simulink model "Dynamic_articulation_FSFA"  (R2018b)
settings: Solver=VariableStepAuto  StartTime=0.0  StopTime=t_final  RelTol=1e-9
values from neighbouring files (symbols this model uses):
  a2 = input(12)    [Nonlinear_model.m]    (also in linear_model.m; linear_model_error.m; trailer_constants.m = 4.98)
  Am = [-0.5 0 0 0 0 0 0 0 ... (first row only)    [Dynamic_model_articulation.m]
  Ap = A    [Dynamic_model_articulation.m]    (also in articulation.m = -1*M_inv*K/u)
  Aprime = A - B1*K    [Dynamic_model_articulation.m]
  B1 = [0,B1(1),0,B1(2),0,B1(3),0,B1(4)]'    [articulation1.m]
  B2 = [0,B2(1),0,B2(2),0,B2(3),0,B2(4)]'    [articulation1.m]
  Bm = [1;0;0;0]    [Dynamic_model_articulation.m]
  Bm2 = B2    [Dynamic_model_articulation.m]
  constants = [C1 C2 C3 m1 m2 I1 I2 a1 l1 h1 b1 a2 l2 Vx]    [Dynamic_model_articulation.m]
  h1 = input(10)    [Nonlinear_model.m]    (also in linear_model.m; linear_model_error.m; truck_constants.m = 1.1)
  K = place(A,B1,Poles)    [FullStateFeedback.m]    (also in articulation.m = [(C+C3),     (Cs1-C3*(h1+l2)+(m1+m2)*u^2),    (-C3*l2),    (; articulation1.m = [(C+C3),     (Cs1-C3*(h1+l2)+(m1+m2)*u^2),    (-C3*l2),    (; linear_model.m = -1/u*K*x_bar; linear_model_error.m = -1/u*K*x_bar)
  Lamda = 0.03    [Dynamic_model_articulation.m]
  Pm = lyap(Am,Q)    [Dynamic_model_articulation.m]
  Vx = 20    [Dynamic_model_articulation.m]
settings Model: Creator=kevingasik  LastModifiedBy=kevingasik
settings DataIOCC: OutputOption=SpecifiedOutputTimes  OutputTimes=[0:0.04:t_final]

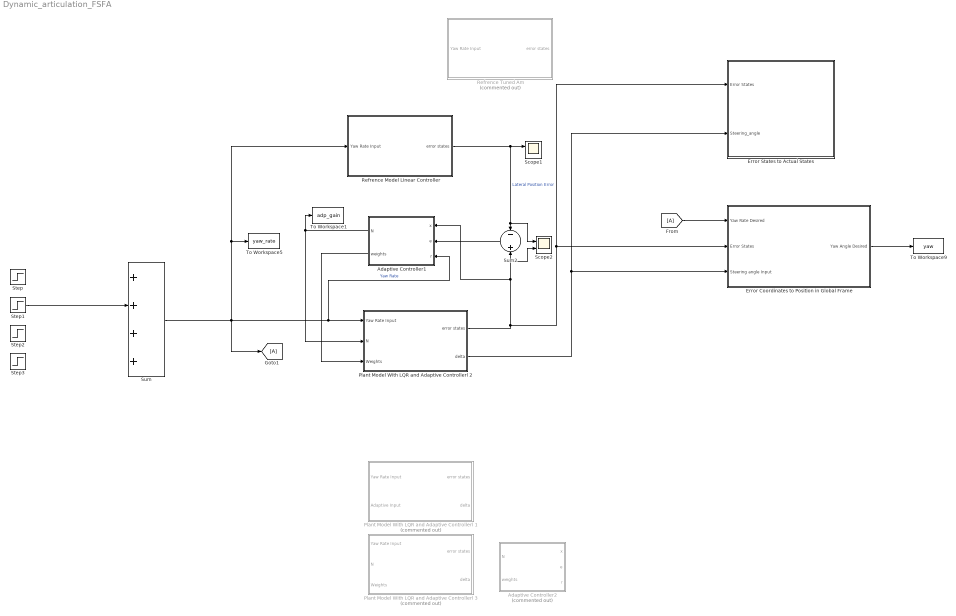
== system Dynamic_articulation_FSFA ==
  Adaptive Controller1 : Subsystem
  Adaptive Controller2 : Subsystem  Commented=on
  "Error Coordinates to Position in Global Frame " : Subsystem
  Error States to Actual States : Subsystem
  Plant Model With LQR and Adaptive Controllerl 1 : Subsystem  Commented=on
  Plant Model With LQR and Adaptive Controllerl 2 : Subsystem
  Plant Model With LQR and Adaptive Controllerl 3 : Subsystem  Commented=on
  Refrence Model Linear Controller : Subsystem
  Refrence Tuned Am : Subsystem  Commented=on
  Scope1 : Scope  NumInputPorts=2
  Scope2 : Scope  NumInputPorts=2
  Step : Step  Time=0  After=0  SampleTime=0
  Step1 : Step  Time=0  After=0.5/180*pi  SampleTime=0
  Step2 : Step  Time=200  After=-1/180*pi  SampleTime=0
  Step3 : Step  Time=110  After=0.5/180*pi  SampleTime=0
  Sum : Sum  Inputs=++++
  Sum2 : Sum  Inputs=-+
  To Workspace1 : ToWorkspace  VariableName=adp_gain  SampleTime=-1
      settings: Save2DSignal=2-D array (concatenate along first dimension)
  To Workspace5 : ToWorkspace  VariableName=yaw_rate  SampleTime=-1
      settings: Save2DSignal=2-D array (concatenate along first dimension)
  To Workspace9 : ToWorkspace  VariableName=yaw  SampleTime=-1
      settings: Save2DSignal=2-D array (concatenate along first dimension)
  wires:
  Sum/1 -> Adaptive Controller1/3(r), Plant Model With LQR and Adaptive Controllerl 2/1(Yaw Rate Input), Refrence Model Linear Controller/1(Yaw Rate Input), To Workspace5/1, [A]  "Yaw Rate"
  Plant Model With LQR and Adaptive Controllerl 2/1(error states) -> "Error Coordinates to Position in Global Frame "/2(Error States), Error States to Actual States/1(Error States), Adaptive Controller1/1(x), Scope2/2, Sum2/2
  Sum2/1 -> Adaptive Controller1/2(e)
  Step1/1 -> Sum/2
  Adaptive Controller1/1(N) -> Plant Model With LQR and Adaptive Controllerl 2/2(N), To Workspace1/1
  [A] -> "Error Coordinates to Position in Global Frame "/1(Yaw Rate Desired)
  Plant Model With LQR and Adaptive Controllerl 2/2(delta) -> Error States to Actual States/2(Steering_angle), "Error Coordinates to Position in Global Frame "/3(Steering angle Input)
  "Error Coordinates to Position in Global Frame "/1(Yaw Angle Desired) -> To Workspace9/1
  Refrence Model Linear Controller/1(error states) -> Scope2/1, Sum2/1, Scope1/1  "Lateral Position Error"
  Adaptive Controller1/2(weights) -> Plant Model With LQR and Adaptive Controllerl 2/3(Weights)

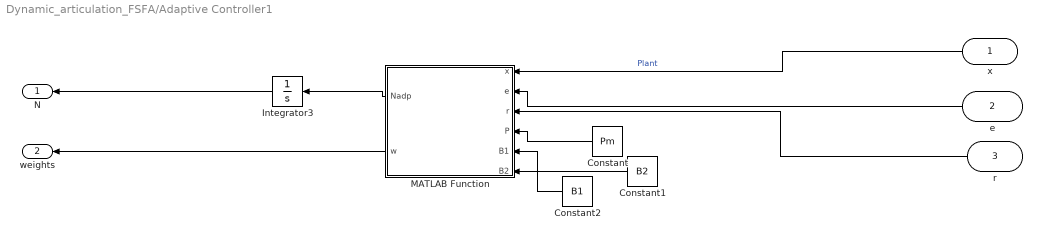
== system Dynamic_articulation_FSFA/Adaptive Controller1 ==
  x : Inport
  e : Inport  Port=2
  r : Inport  Port=3
  Constant : Constant  Value=Pm  VectorParams1D=off
  Constant1 : Constant  Value=B2  VectorParams1D=off
  Constant2 : Constant  Value=B1  VectorParams1D=off
  Integrator3 : Integrator  InitialCondition=[0 0 0 0 0 0 0 0 0 0]
  MATLAB Function : MATLAB Function  TreatAsAtomicUnit=on
  N : Outport
  weights : Outport  Port=2
  wires:
  r/1 -> MATLAB Function/3(r)
  MATLAB Function/2(w) -> weights/1
  Constant/1 -> MATLAB Function/4(P)
  x/1 -> MATLAB Function/1(x)  "Plant"
  Integrator3/1 -> N/1
  MATLAB Function/1(Nadp) -> Integrator3/1
  e/1 -> MATLAB Function/2(e)
  Constant2/1 -> MATLAB Function/5(B1)
  Constant1/1 -> MATLAB Function/6(B2)

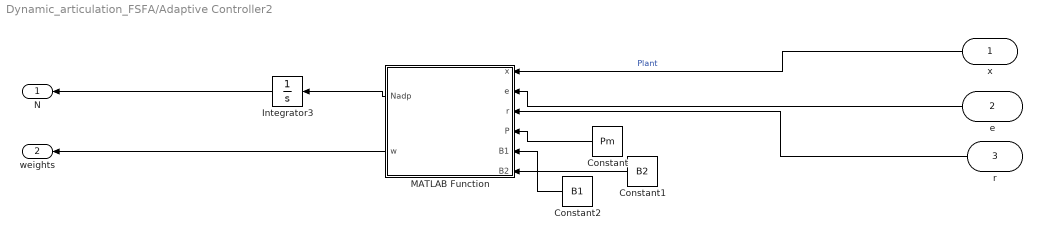
== system Dynamic_articulation_FSFA/Adaptive Controller2 ==
  x : Inport
  e : Inport  Port=2
  r : Inport  Port=3
  Constant : Constant  Value=Pm  VectorParams1D=off
  Constant1 : Constant  Value=B2  VectorParams1D=off
  Constant2 : Constant  Value=B1  VectorParams1D=off
  Integrator3 : Integrator  InitialCondition=[0 0 0 0 0 0 0 0 0 0]
  MATLAB Function : MATLAB Function  TreatAsAtomicUnit=on
  N : Outport
  weights : Outport  Port=2
  wires:
  r/1 -> MATLAB Function/3(r)
  MATLAB Function/2(w) -> weights/1
  Constant/1 -> MATLAB Function/4(P)
  x/1 -> MATLAB Function/1(x)  "Plant"
  Integrator3/1 -> N/1
  MATLAB Function/1(Nadp) -> Integrator3/1
  e/1 -> MATLAB Function/2(e)
  Constant2/1 -> MATLAB Function/5(B1)
  Constant1/1 -> MATLAB Function/6(B2)

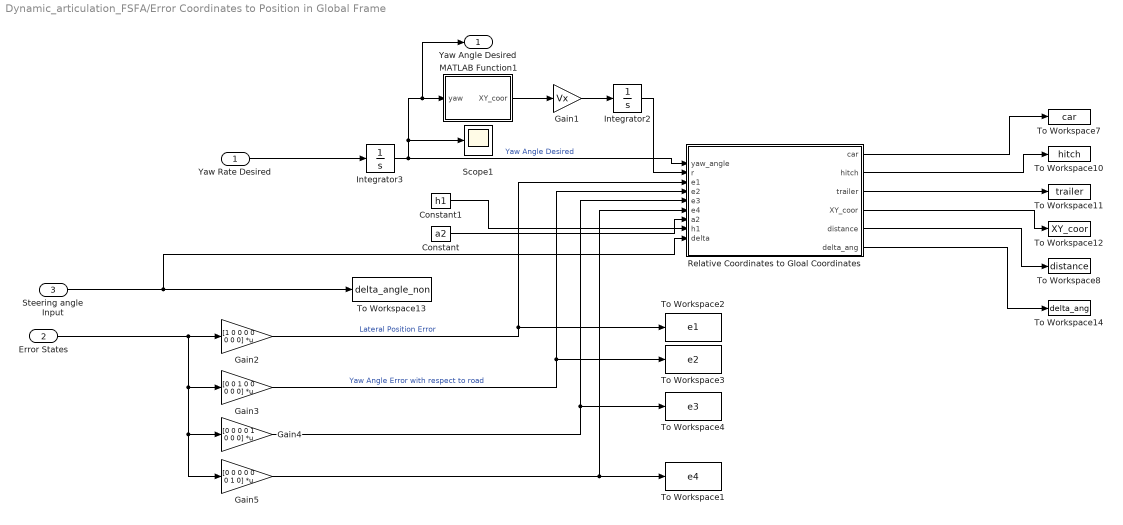
== system Dynamic_articulation_FSFA/Error Coordinates to Position in Global Frame  ==
  Yaw Rate Desired : Inport
  Error States : Inport  Port=2
  Steering angle Input : Inport  Port=3
  Constant : Constant  Value=a2
  Constant1 : Constant  Value=h1
  Gain1 : Gain  Gain=Vx
  Gain2 : Gain  Gain=[1 0 0 0 0 0 0 0]  Multiplication=Matrix(K*u)
  Gain3 : Gain  Gain=[0 0 1 0 0 0 0 0]  Multiplication=Matrix(K*u)
  Gain4 : Gain  Gain=[0 0 0 0 1 0 0 0]  Multiplication=Matrix(K*u)
  Gain5 : Gain  Gain=[0 0 0 0 0 0 1 0]  Multiplication=Matrix(K*u)
  Integrator2 : Integrator
  Integrator3 : Integrator
  MATLAB Function1 : MATLAB Function  TreatAsAtomicUnit=on
  Relative Coordinates to Gloal Coordinates : MATLAB Function  TreatAsAtomicUnit=on
  Scope1 : Scope
  To Workspace1 : ToWorkspace  VariableName=e4  SampleTime=-1
      settings: Save2DSignal=2-D array (concatenate along first dimension)
  To Workspace10 : ToWorkspace  VariableName=hitch  SampleTime=-1
      settings: Save2DSignal=2-D array (concatenate along first dimension)
  To Workspace11 : ToWorkspace  VariableName=trailer  SampleTime=-1
      settings: Save2DSignal=2-D array (concatenate along first dimension)
  To Workspace12 : ToWorkspace  VariableName=XY_coor  SampleTime=-1
      settings: Save2DSignal=2-D array (concatenate along first dimension)
  To Workspace13 : ToWorkspace  VariableName=delta_angle_non  SampleTime=-1
      settings: Save2DSignal=2-D array (concatenate along first dimension)
  To Workspace14 : ToWorkspace  VariableName=delta_ang  SampleTime=-1
      settings: Save2DSignal=2-D array (concatenate along first dimension)
  To Workspace2 : ToWorkspace  VariableName=e1  SampleTime=-1
      settings: Save2DSignal=2-D array (concatenate along first dimension)
  To Workspace3 : ToWorkspace  VariableName=e2  SampleTime=-1
      settings: Save2DSignal=2-D array (concatenate along first dimension)
  To Workspace4 : ToWorkspace  VariableName=e3  SampleTime=-1
      settings: Save2DSignal=2-D array (concatenate along first dimension)
  To Workspace7 : ToWorkspace  VariableName=car  SampleTime=-1
      settings: Save2DSignal=2-D array (concatenate along first dimension)
  To Workspace8 : ToWorkspace  VariableName=distance  SampleTime=-1
      settings: Save2DSignal=2-D array (concatenate along first dimension)
  Yaw Angle Desired : Outport
  wires:
  Relative Coordinates to Gloal Coordinates/4(XY_coor) -> To Workspace12/1
  Yaw Rate Desired/1 -> Integrator3/1
  Relative Coordinates to Gloal Coordinates/3(trailer) -> To Workspace11/1
  MATLAB Function1/1(XY_coor) -> Gain1/1
  Gain2/1 -> Relative Coordinates to Gloal Coordinates/3(e1), To Workspace2/1  "Lateral Position Error"
  Relative Coordinates to Gloal Coordinates/6(delta_ang) -> To Workspace14/1
  Steering angle Input/1 -> To Workspace13/1, Relative Coordinates to Gloal Coordinates/9(delta)
  Gain5/1 -> Relative Coordinates to Gloal Coordinates/6(e4), To Workspace1/1
  Constant1/1 -> Relative Coordinates to Gloal Coordinates/8(h1)
  Relative Coordinates to Gloal Coordinates/5(distance) -> To Workspace8/1
  Relative Coordinates to Gloal Coordinates/2(hitch) -> To Workspace10/1
  Integrator2/1 -> Relative Coordinates to Gloal Coordinates/2(r)
  Integrator3/1 -> Yaw Angle Desired/1, MATLAB Function1/1(yaw), Scope1/1, Relative Coordinates to Gloal Coordinates/1(yaw_angle)  "Yaw Angle Desired"
  Constant/1 -> Relative Coordinates to Gloal Coordinates/7(a2)
  Error States/1 -> Gain3/1, Gain4/1, Gain5/1, Gain2/1
  Gain4/1 -> Relative Coordinates to Gloal Coordinates/5(e3), To Workspace4/1
  Gain1/1 -> Integrator2/1
  Relative Coordinates to Gloal Coordinates/1(car) -> To Workspace7/1
  Gain3/1 -> To Workspace3/1, Relative Coordinates to Gloal Coordinates/4(e2)  "Yaw Angle Error with respect to road"

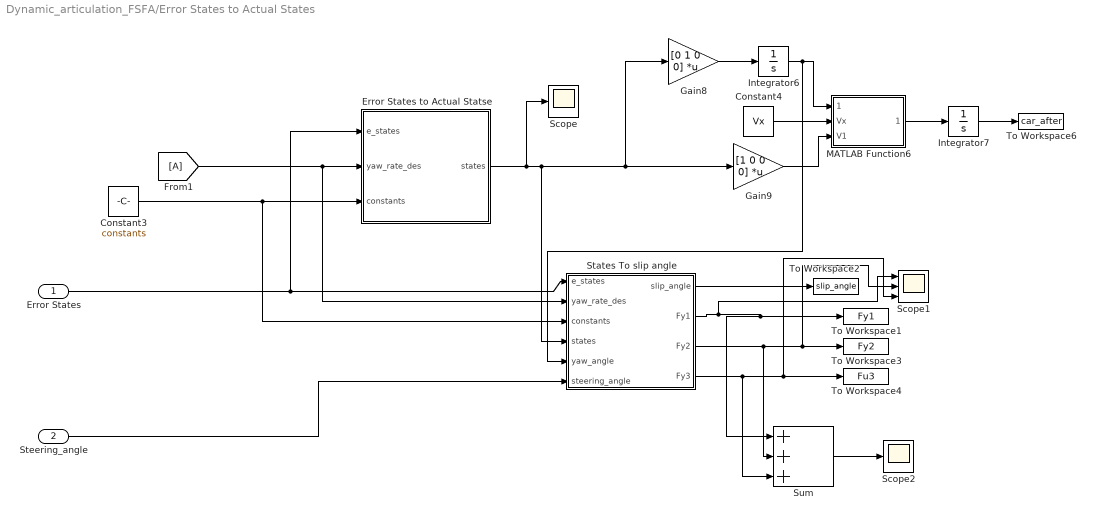
== system Dynamic_articulation_FSFA/Error States to Actual States ==
  Error States : Inport
  Steering_angle : Inport  Port=2
  Constant3 : Constant  Value=constants
  Constant4 : Constant  Value=Vx
  Error States to Actual Statse : MATLAB Function  TreatAsAtomicUnit=on
  Gain8 : Gain  Gain=[0 1 0 0]  Multiplication=Matrix(K*u)
  Gain9 : Gain  Gain=[1 0 0 0]  Multiplication=Matrix(K*u)
  Integrator6 : Integrator
  Integrator7 : Integrator
  MATLAB Function6 : MATLAB Function  TreatAsAtomicUnit=on
  Scope : Scope
  Scope1 : Scope  NumInputPorts=3
  Scope2 : Scope
  States To slip angle : MATLAB Function  TreatAsAtomicUnit=on
  Sum : Sum  Inputs=+++
  To Workspace1 : ToWorkspace  VariableName=Fy1  SampleTime=-1
      settings: Save2DSignal=2-D array (concatenate along first dimension)
  To Workspace2 : ToWorkspace  VariableName=slip_angle  SampleTime=-1
      settings: Save2DSignal=2-D array (concatenate along first dimension)
  To Workspace3 : ToWorkspace  VariableName=Fy2  SampleTime=-1
      settings: Save2DSignal=2-D array (concatenate along first dimension)
  To Workspace4 : ToWorkspace  VariableName=Fu3  SampleTime=-1
      settings: Save2DSignal=2-D array (concatenate along first dimension)
  To Workspace6 : ToWorkspace  VariableName=car_after  SampleTime=-1
      settings: Save2DSignal=2-D array (concatenate along first dimension)
  wires:
  Constant3/1 -> States To slip angle/3(constants), Error States to Actual Statse/3(constants)
  Gain9/1 -> MATLAB Function6/3(V1)
  MATLAB Function6/1(XY_coor) -> Integrator7/1
  Error States/1 -> States To slip angle/1(e_states), Error States to Actual Statse/1(e_states)
  Constant4/1 -> MATLAB Function6/2(Vx)
  Error States to Actual Statse/1(states) -> Scope/1, States To slip angle/4(states), Gain9/1, Gain8/1
  Gain8/1 -> Integrator6/1
  Integrator7/1 -> To Workspace6/1
  [A] -> States To slip angle/2(yaw_rate_des), Error States to Actual Statse/2(yaw_rate_des)
  Steering_angle/1 -> States To slip angle/6(steering_angle)
  Integrator6/1 -> States To slip angle/5(yaw_angle), MATLAB Function6/1(yaw_angle)
  States To slip angle/1(slip_angle) -> To Workspace2/1
  States To slip angle/2(Fy1) -> To Workspace1/1, Sum/1, Scope1/1
  States To slip angle/3(Fy2) -> Sum/2, Scope1/2, To Workspace3/1
  States To slip angle/4(Fy3) -> Sum/3, Scope1/3, To Workspace4/1
  Sum/1 -> Scope2/1

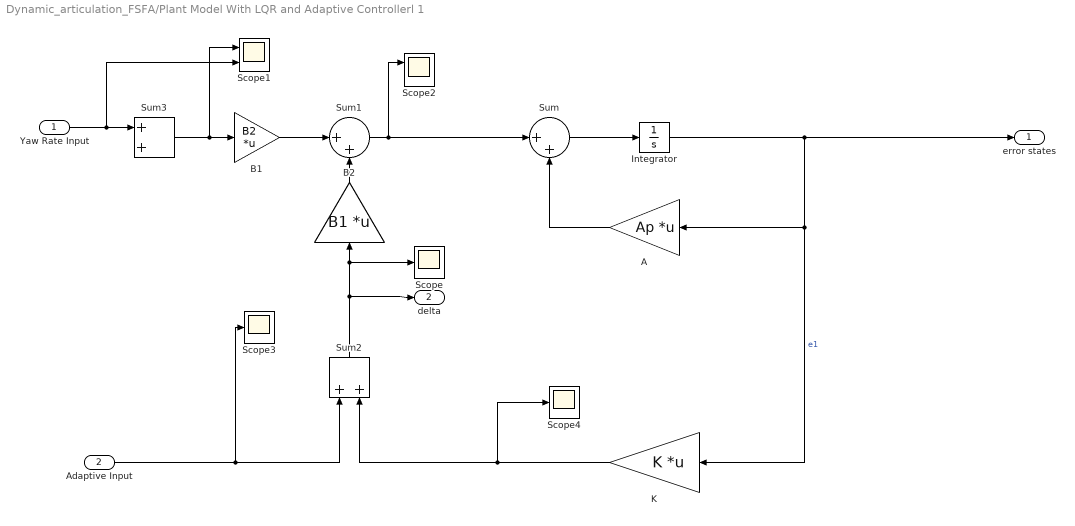
== system Dynamic_articulation_FSFA/Plant Model With LQR and Adaptive Controllerl 1 ==
  Yaw Rate Input : Inport
  Adaptive Input : Inport  Port=2
  A : Gain  Gain=Ap  Multiplication=Matrix(K*u)
  B1 : Gain  Gain=B2  Multiplication=Matrix(K*u)
  B2 : Gain  Gain=B1  Multiplication=Matrix(K*u)
  Integrator : Integrator
  K : Gain  Gain=K  Multiplication=Matrix(K*u)
  Scope : Scope
  Scope1 : Scope  NumInputPorts=2
  Scope2 : Scope  NumInputPorts=2
  Scope3 : Scope
  Scope4 : Scope
  Sum : Sum  Inputs=|++
  Sum1 : Sum  Inputs=|++
  Sum2 : Sum
  Sum3 : Sum
  error states : Outport
  delta : Outport  Port=2
  wires:
  Sum/1 -> Integrator/1
  A/1 -> Sum/2
  Integrator/1 -> error states/1, K/1, A/1  "e1"
  B1/1 -> Sum1/1
  B2/1 -> Sum1/2
  Sum1/1 -> Scope2/1, Sum/1
  Yaw Rate Input/1 -> Scope1/2, Sum3/1
  Sum3/1 -> B1/1, Scope1/1
  K/1 -> Scope4/1, Sum2/2
  Adaptive Input/1 -> Scope3/1, Sum2/1
  Sum2/1 -> Scope/1, B2/1, delta/1

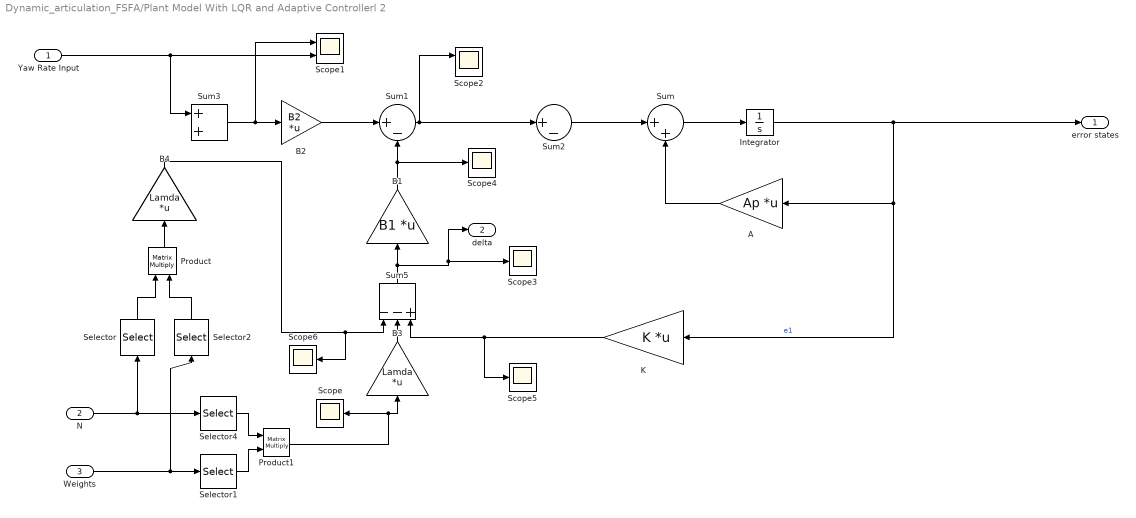
== system Dynamic_articulation_FSFA/Plant Model With LQR and Adaptive Controllerl 2 ==
  Yaw Rate Input : Inport
  N : Inport  Port=2
  Weights : Inport  Port=3
  A : Gain  Gain=Ap  Multiplication=Matrix(K*u)
  B1 : Gain  Gain=B1  Multiplication=Matrix(K*u)
  B2 : Gain  Gain=B2  Multiplication=Matrix(K*u)
  B3 : Gain  Gain=Lamda  Multiplication=Matrix(K*u)
  B4 : Gain  Gain=Lamda  Multiplication=Matrix(K*u)
  Integrator : Integrator
  K : Gain  Gain=K  Multiplication=Matrix(K*u)
  Product : Product  Multiplication=Matrix(*)
  Product1 : Product  Multiplication=Matrix(*)
  Scope{,3..6} (5 alike) : Scope
  Scope1 : Scope  NumInputPorts=2
  Scope2 : Scope  NumInputPorts=2
  Selector : Selector  InputPortWidth=10  IndexOptions=Index vector (dialog)  Indices=[10]  OutputSizes=1
  Selector1 : Selector  InputPortWidth=10  IndexOptions=Index vector (dialog)  Indices=[1 2 3 4 5 6 7 8 ]  OutputSizes=1
  Selector2 : Selector  InputPortWidth=10  IndexOptions=Index vector (dialog)  Indices=[10]  OutputSizes=1
  Selector4 : Selector  InputPortWidth=10  IndexOptions=Index vector (dialog)  Indices=[1 2 3 4 5 6 7 8 ]  OutputSizes=1
  Sum : Sum  Inputs=|++
  Sum1 : Sum  Inputs=|+-
  Sum2 : Sum  Inputs=|+-
  Sum3 : Sum
  Sum5 : Sum  Inputs=--+
  error states : Outport
  delta : Outport  Port=2
  wires:
  Sum/1 -> Integrator/1
  A/1 -> Sum/2
  B2/1 -> Sum1/1
  Selector/1 -> Product/1
  Selector2/1 -> Product/2
  Integrator/1 -> error states/1, K/1, A/1  "e1"
  K/1 -> Sum5/3, Scope5/1
  Sum1/1 -> Scope2/1, Sum2/1
  B1/1 -> Sum1/2, Scope4/1
  Yaw Rate Input/1 -> Sum3/1, Scope1/2
  Sum2/1 -> Sum/1
  Sum3/1 -> Scope1/1, B2/1
  Product1/1 -> B3/1, Scope/1
  Sum5/1 -> Scope3/1, delta/1, B1/1
  N/1 -> Selector4/1, Selector/1
  Weights/1 -> Selector1/1, Selector2/1
  Selector4/1 -> Product1/1
  Product/1 -> B4/1
  Selector1/1 -> Product1/2
  B3/1 -> Sum5/2
  B4/1 -> Scope6/1, Sum5/1

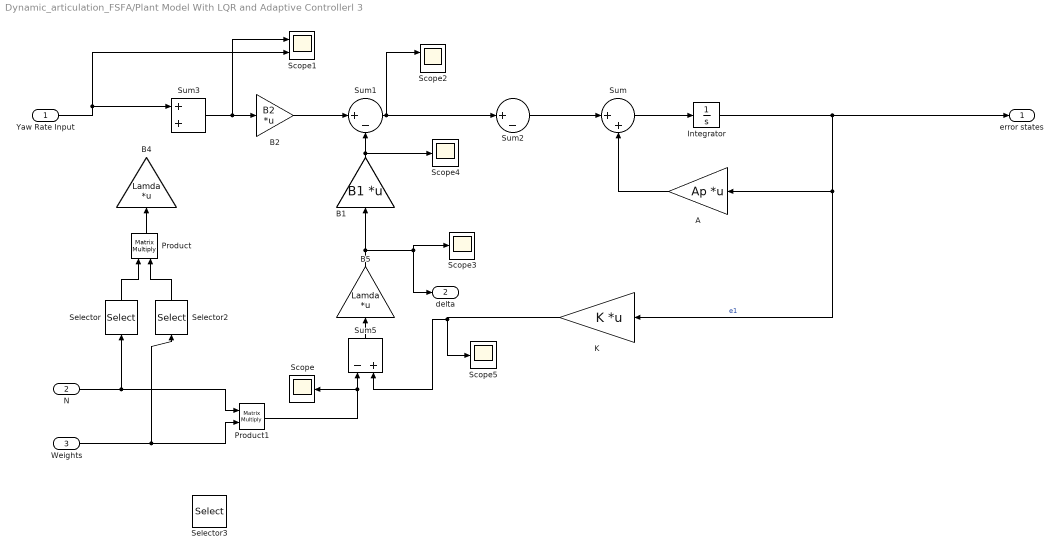
== system Dynamic_articulation_FSFA/Plant Model With LQR and Adaptive Controllerl 3 ==
  Yaw Rate Input : Inport
  N : Inport  Port=2
  Weights : Inport  Port=3
  A : Gain  Gain=Ap  Multiplication=Matrix(K*u)
  B1 : Gain  Gain=B1  Multiplication=Matrix(K*u)
  B2 : Gain  Gain=B2  Multiplication=Matrix(K*u)
  B4 : Gain  Gain=Lamda  Multiplication=Matrix(K*u)
  B5 : Gain  Gain=Lamda  Multiplication=Matrix(K*u)
  Integrator : Integrator
  K : Gain  Gain=K  Multiplication=Matrix(K*u)
  Product : Product  Multiplication=Matrix(*)
  Product1 : Product  Multiplication=Matrix(*)
  Scope{,3..5} (4 alike) : Scope
  Scope1 : Scope  NumInputPorts=2
  Scope2 : Scope  NumInputPorts=2
  Selector : Selector  InputPortWidth=10  IndexOptions=Index vector (dialog)  Indices=[10]  OutputSizes=1
  Selector2 : Selector  InputPortWidth=10  IndexOptions=Index vector (dialog)  Indices=[10]  OutputSizes=1
  Selector3 : Selector  InputPortWidth=10  IndexOptions=Index vector (dialog)  Indices=[1 2 3 4 5 6 7 8 ]  OutputSizes=1
  Sum : Sum  Inputs=|++
  Sum1 : Sum  Inputs=|+-
  Sum2 : Sum  Inputs=|+-
  Sum3 : Sum
  Sum5 : Sum  Inputs=-+
  error states : Outport
  delta : Outport  Port=2
  wires:
  Sum/1 -> Integrator/1
  A/1 -> Sum/2
  B2/1 -> Sum1/1
  Selector/1 -> Product/1
  Selector2/1 -> Product/2
  Integrator/1 -> error states/1, K/1, A/1  "e1"
  K/1 -> Sum5/2, Scope5/1
  Sum1/1 -> Scope2/1, Sum2/1
  B1/1 -> Sum1/2, Scope4/1
  Yaw Rate Input/1 -> Sum3/1, Scope1/2
  Sum2/1 -> Sum/1
  Sum3/1 -> Scope1/1, B2/1
  Sum5/1 -> B5/1
  Product1/1 -> Scope/1, Sum5/1
  N/1 -> Product1/1, Selector/1
  Product/1 -> B4/1
  Weights/1 -> Product1/2, Selector2/1
  B5/1 -> delta/1, Scope3/1, B1/1

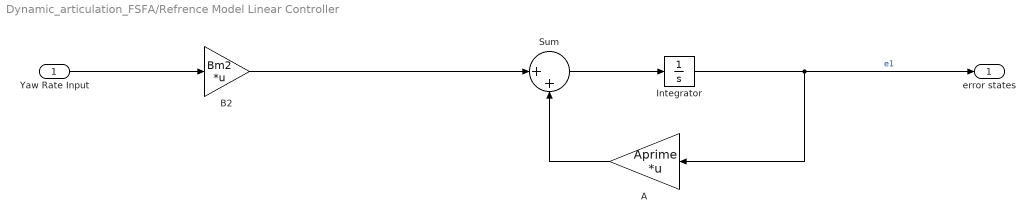
== system Dynamic_articulation_FSFA/Refrence Model Linear Controller ==
  Yaw Rate Input : Inport
  A : Gain  Gain=Aprime  Multiplication=Matrix(K*u)
  B2 : Gain  Gain=Bm2  Multiplication=Matrix(K*u)
  Integrator : Integrator
  Sum : Sum  Inputs=|++
  error states : Outport
  wires:
  Sum/1 -> Integrator/1
  A/1 -> Sum/2
  Integrator/1 -> A/1, error states/1  "e1"
  Yaw Rate Input/1 -> B2/1
  B2/1 -> Sum/1

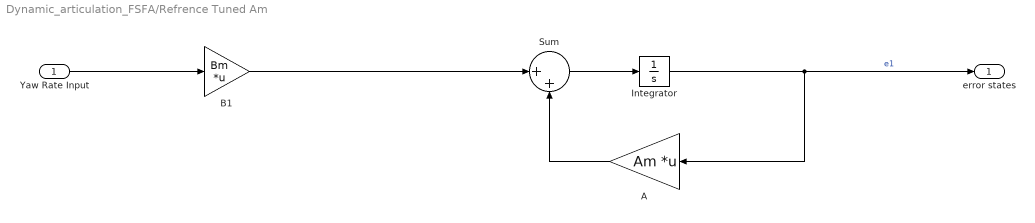
== system Dynamic_articulation_FSFA/Refrence Tuned Am ==
  Yaw Rate Input : Inport
  A : Gain  Gain=Am  Multiplication=Matrix(K*u)
  B1 : Gain  Gain=Bm  Multiplication=Matrix(K*u)
  Integrator : Integrator
  Sum : Sum  Inputs=|++
  error states : Outport
  wires:
  Sum/1 -> Integrator/1
  A/1 -> Sum/2
  Integrator/1 -> error states/1, A/1  "e1"
  Yaw Rate Input/1 -> B1/1
  B1/1 -> Sum/1

== matlab function Dynamic_articulation_FSFA/Error Coordinates to Position in Global Frame /Relative Coordinates to Gloal Coordinates ==
  data: yaw_angle input; r input; e1 input; car output; hitch output; trailer output; XY_coor output; e2 input; e3 input; e4 input; a2 input; h1 input; distance output; delta input; delta_ang output
function [car,hitch,trailer,XY_coor,distance,delta_ang] = fcn(yaw_angle,r,e1,e2,e3, e4, a2,h1,delta)
XY_coor = [0 0];
trailer = [0 0];
hitch = [0 0];
car = [0 0];
angle = 0;
delta_ang = 0;
XY_dot_coor = [0 0];


%%Transformation matrices from local to global coordinates
Q = [-sin(yaw_angle+e2),cos(yaw_angle+e2)];
R = [-cos(yaw_angle+e2),-sin(yaw_angle+e2)];
T = [-cos(yaw_angle+e4),-sin(yaw_angle+e4)];

%% desired trajectory
X_des = r(1,1);
Y_des = r(1,2);
%X_des2 = r(1,1) - (a2+h1)*cosd(yaw_angle+e2);
%Y_des2 = r(1,2) - (a2+h1)*sind(yaw_angle+e2);
XY_coor = [X_des,Y_des];

%outputting the correct output.
car_x = r(1,1)+ e1*Q(1,1);
car_y = r(1,2)+ e1*Q(1,2);
car = [car_x,car_y];

hitch_x = r(1,1) + e1*Q(1,1) + h1*R(1,1);
hitch_y = r(1,2) + e1*Q(1,2) + h1*R(1,2);
%hitch_a = X_des2 + e3*Q(1,1) - a2*T(1,1);
%hitch_b = Y_des2 + e3*Q(1,2) - a2*T(1,2);
hitch = [hitch_x,hitch_y];


trailer_x = r(1,1)+ (e1)*Q(1,1) + h1*R(1,1) + a2*T(1,1);
trailer_y = r(1,2)+ (e1)*Q(1,2) + h1*R(1,2) + a2*T(1,2);
%trailer_x = X_des2 + e3*Q(1,1);
%trailer_y = Y_des2 + e3*Q(1,2);


distance = sqrt((abs(hitch_x-trailer_x))^2 + abs(hitch_y-trailer_y)^2);
delta_ang = delta + e2 + yaw_angle; 
trailer = [trailer_x,trailer_y];

== matlab function Dynamic_articulation_FSFA/Error Coordinates to Position in Global Frame /MATLAB Function1 ==
  data: yaw input; XY_coor output
function XY_coor  = fcn(yaw)

XY_coor = [cos(yaw),sin(yaw)];

== matlab function Dynamic_articulation_FSFA/Error States to Actual States/Error States to Actual Statse ==
  data: e_states input; yaw_rate_des input; constants input; states output
function states = fcn(e_states,yaw_rate_des,constants)

states = [0;0;0;0];

a2 = constants(12);
u =  constants(14);

e = [e_states(1) e_states(3) e_states(5) e_states(7)]';
ed = [e_states(2) e_states(4) e_states(6) e_states(8)]';


p1 = [1,        0,              0,      0;
      0,        1,              0,      0;
      1/a2,     0,           -1/a2,     0;  
      0,        0,              0,      0];
                
p2 = [0,        -u,      0,      0;
      0,         0,      0,      0;
      0,     -u/a2,      0,   u/a2;
      0,        -1,      0,      1]; %% phi = -e2 + e4
               
p3 = [0;1;0;0]; % \dot \psi desired 

states = p1*ed + p2*e + p3*yaw_rate_des;

== matlab function Dynamic_articulation_FSFA/Error States to Actual States/States To slip angle ==
  data: e_states input; yaw_rate_des input; constants input; slip_angle output; states input; yaw_angle input; steering_angle input; Fy1 output; Fy2 output; Fy3 output
function [slip_angle,Fy1,Fy2,Fy3] = fcn(e_states,yaw_rate_des,constants,states,yaw_angle,steering_angle)

slip_angle = 0;

C1 = constants(1);
C2 = constants(2);
C3 = constants(3);
a1 = constants(8);
h1 = constants(10);
b1 = constants(11);
a2 = constants(12);
l2 = constants(13);
u =  constants(14);

e = [e_states(1) e_states(3) e_states(5) e_states(7)]';
ed = [e_states(2) e_states(4) e_states(6) e_states(8)]';


slip_angle = steering_angle - states(2)*a1/u - yaw_angle;
%slip_angle = 1/20*(ed(1))-e(2);
Fy1 = -1/u*C1*(states(1) + a1*states(2)) + C1*steering_angle
Fy2 = -1/u*C2*(states(1) - b1*states(2))
Fy3 = -1/u*C3*(states(1) - h1*states(2) - l2*states(3))+C3*steering_angle

== matlab function Dynamic_articulation_FSFA/Adaptive Controller1/MATLAB Function ==
  data: x input; Nadp output; e input; r input; P input; w output; B1 input; B2 input
function [Nadp,w]   = fcn(x,e,r,P,B1,B2)

w = [0;0;0;0;0;0;0;0;0;0];
Nadp = [0;0;0;0;0;0;0;0;0;0]';

%x = [10*x(1); x(2);0;x(4);0;0;0;0];
%e = [10*e(1); e(2);0;e(4);0;0;0;0];
%x = [x(1); x(2);x(3);x(4);x(5);x(6);x(7);x(8)];
%e = [10*e(1); e(2);e(3);e(4);10*e(5);e(6);120*e(7);120*e(8)];
x = [x(1); x(2);x(3);x(4);x(5);x(6);x(7);x(8)];
e = [18*e(1); 118*e(2);e(3);15*e(4);155*e(5);e(6);220*e(7);12*e(8)];


%% define learning rate
gr = 1; 
gx = (eye(8));
ydd = 1;

%% Thesis paper
%w = 1*[0.0001*x' ydd r]';
w = 0.0001*[x' ydd r]';

theta_xd = -gx*x*e'*P*B1;
theta_d_d = -ydd*e'*P*B1;

if(e'*e <= 0.0001)
    theta_rd = 0;
    theta_xd = [0 0 0 0 0 0 0 0]';
    theta_d_d = 0;
else( e'*e >= 0.0001) 
    %theta_rd = -gr*e'*P*B2;
    theta_rd = -gr*e'*P*B1;
    theta_xd = -gx*x*e'*P*B1;
    theta_d_d = 0;
end

Nadp = [theta_xd' theta_d_d' theta_rd']

== matlab function Dynamic_articulation_FSFA/Adaptive Controller2/MATLAB Function ==
  data: x input; Nadp output; e input; r input; P input; w output; B1 input; B2 input
function [Nadp,w]   = fcn(x,e,r,P,B1,B2)

w = [0;0;0;0;0;0;0;0;0;0];
Nadp = [0;0;0;0;0;0;0;0;0;0]';

%x = [0; 0;0;0;0;0;0;x(8)];
%e = [0; 0;0;0;0;0;0;e(8)];

%% define learning rate
gr = 1; 
gx = (eye(8));
ydd = 1;

%% Thesis paper
w = 0.00001*[x' ydd r]';

if(e'*e <= 0.005)
     theta_xd = [0 0 0 0 0 0 0 0]';
     theta_rd = 0;
     theta_d_d = 0;
    
else(e'*e >= 0.005) 
    theta_rd = -gr*e'*P*B1;
    %theta_rd = 0;
    %theta_d_d = 0;
    theta_xd = -gx*x*e'*P*B1;
    theta_d_d = -ydd*e'*P*B1;
end

Nadp = [theta_xd' theta_d_d' theta_rd']

== matlab function Dynamic_articulation_FSFA/Error States to Actual States/MATLAB Function6 ==
  data: yaw_angle input; XY_coor output; Vx input; V1 input
function XY_coor  = fcn(yaw_angle,Vx,V1)

XY_coor = [(Vx*cos(yaw_angle) - V1*sin(yaw_angle)),(V1*cos(yaw_angle) + Vx*sin(yaw_angle))];
%xdot = XY_coor(1);
%ydot = XY_coor(2);

%xdot_p = xdot*cos(yaw_angle) - ydot*sin(yaw_angle); 
%ydot_p = xdot*sin(yaw_angle) + ydot*cos(yaw_angle);

%XY_coor = [xdot_p, ydot_p];
